simulink model "simulink_pi"  (R2018a)
settings: Solver=VariableStepAuto  StartTime=0.0  StopTime=500  RelTol=1e-3
values from neighbouring files (symbols this model uses):
  ae = 329.2  / fator    (= 5.48666666667)    [carregaDadosDoModelo.m]    (also in carregaDadosSimulacao.m = 5.4867)
  anp = 16.5    [carregaDadosSimulacao.m]
  av = 414.17 / fator    (= 6.90283333333)    [carregaDadosDoModelo.m]    (also in carregaDadosSimulacao.m = 6.9028)
  K = 0.36783    [carregaDados.m]    (also in carregaDadosDoModelo.m = 0.01332; carregaDadosSimulacao.m = 0.01)
  Kc = 1       * fator    (= 60)    [carregaDadosDoModelo.m]    (also in carregaDadosSimulacao.m = 2.5)
  Ke = 0.395   * fator    (= 23.7)    [carregaDadosDoModelo.m]    (also in carregaDadosSimulacao.m = 1.4)
  Ki = 13 * Kp    (= 1.56)    [carregaDados.m]    (also in carregaDadosSimulacao.m)
  Knp = 0.1    [carregaDadosSimulacao.m]
  Kp = 0.12    [carregaDados.m]    (also in carregaDadosSimulacao.m)
  Kpwm = 20    [carregaDadosSimulacao.m]
  Kr = 0.016835* fator    (= 1.0101)    [carregaDadosDoModelo.m]
  Ktp = 36.5    [carregaDadosSimulacao.m]
  Kv = 0.647   * fator    (= 38.82)    [carregaDadosDoModelo.m]    (also in carregaDadosSimulacao.m = 3.3)
  td = 0.065    [carregaDados.m]    (also in carregaDadosSimulacao.m = 5)
settings Model: Creator=alexa  LastModifiedBy=alexa

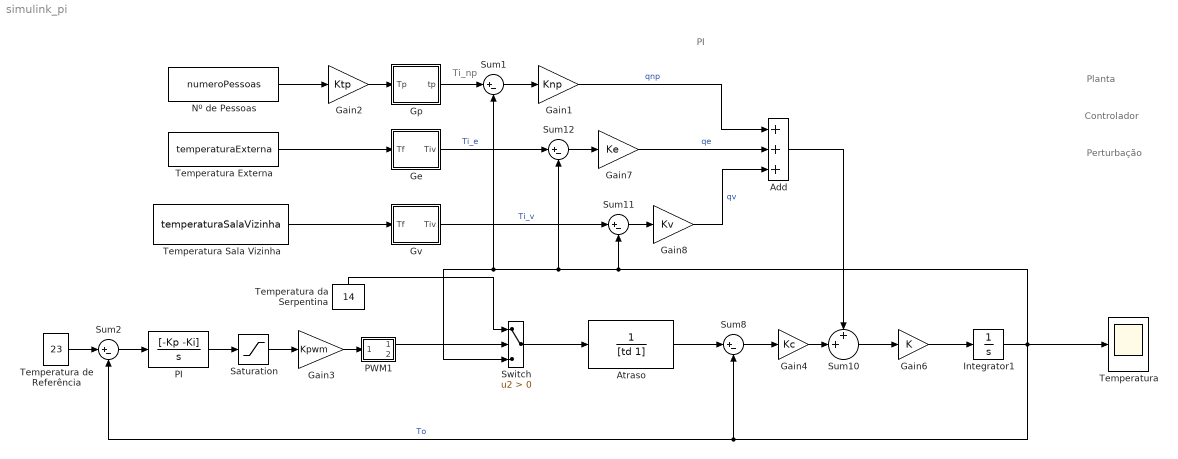
== system simulink_pi ==
  note: Planta
  note: Perturbação
  note: Ti_np
  note: Controlador
  note: PI
  Add : Sum  Inputs=+++
  Atraso : TransferFcn  Denominator=[td 1]
  Gain1 : Gain  Gain=Knp
  Gain2 : Gain  Gain=Ktp
  Gain3 : Gain  Gain=Kpwm
  Gain4 : Gain  Gain=Kc
  Gain6 : Gain  Gain=K
  Gain7 : Gain  Gain=Ke
  Gain8 : Gain  Gain=Kv
  Ge : Subsystem
  Gp : Subsystem
  Gv : Subsystem
  Integrator1 : Integrator  InitialCondition=24
  Nº de Pessoas : FromWorkspace  VariableName=numeroPessoas  SampleTime=1
  PI : TransferFcn  Numerator=[-Kp -Ki]  Denominator=[1 0]
  PWM1 : Subsystem  mask(Pulse Generator){period=1, amplitude=1, start=0}
      mask prompts: period "Period (secs):"; start "Start time:"
      mask help: Pulse Generator
      mask Help: Pulse generator which ensures pulse transitions are hit. Provides a vector of pulses when the height is entered as a vector.  Unmask to see how it works.
      mask Display: plot(0,0,100,100,[95,90,90,75,75,60,60,45,45,30,30,15,15,5],[25,25,75,75,25,25,75,75,25,25,75,75,25,25]);
  Saturation : Saturate  UpperLimit=0.05  LowerLimit=-0.05
  Sum{1..2,8,11..12} (5 alike) : Sum  Inputs=|+-
  Sum10 : Sum  Inputs=++|
  Switch : Switch  Criteria=u2 > Threshold
  Temperatura : Scope
  Temperatura da Serpentina : Constant  Value=14
  Temperatura de Referência : Constant  Value=23
  Temperatura Externa : FromWorkspace  VariableName=temperaturaExterna  SampleTime=1
  Temperatura Sala Vizinha : FromWorkspace  VariableName=temperaturaSalaVizinha  SampleTime=1
  wires:
  Sum12/1 -> Gain7/1
  Sum8/1 -> Gain4/1
  Gain7/1 -> Add/2  "qe"
  Gain2/1 -> Gp/1(Tp)
  Nº de Pessoas/1 -> Gain2/1
  Gp/1("tp ") -> Sum1/1
  Gain8/1 -> Add/3  "qv"
  Gain1/1 -> Add/1  "qnp"
  Temperatura Externa/1 -> Ge/1(Tf)
  Ge/1(Tiv) -> Sum12/1  "Ti_e"
  Integrator1/1 -> Temperatura/1, Sum8/2, Sum2/2, Switch/3, Sum1/2, Sum12/2, Sum11/2  "To"
  Temperatura da Serpentina/1 -> Switch/1
  Temperatura Sala Vizinha/1 -> Gv/1(Tf)
  Switch/1 -> Atraso/1
  Add/1 -> Sum10/1
  Gv/1(Tiv) -> Sum11/1  "Ti_v"
  Atraso/1 -> Sum8/1
  Sum11/1 -> Gain8/1
  Gain6/1 -> Integrator1/1
  Sum1/1 -> Gain1/1
  Sum10/1 -> Gain6/1
  Gain4/1 -> Sum10/2
  Temperatura de Referência/1 -> Sum2/1
  Sum2/1 -> PI/1
  PI/1 -> Saturation/1
  PWM1/1(Out1) -> Switch/2
  Saturation/1 -> Gain3/1
  Gain3/1 -> PWM1/1(In1)

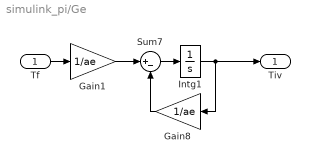
== system simulink_pi/Ge ==
  Tf : Inport
  Gain1 : Gain  Gain=1/ae
  Gain8 : Gain  Gain=1/ae
  Intg1 : Integrator  InitialCondition=30
  Sum7 : Sum  Inputs=|+-
  Tiv : Outport
  wires:
  Gain1/1 -> Sum7/1
  Tf/1 -> Gain1/1
  Gain8/1 -> Sum7/2
  Intg1/1 -> Tiv/1, Gain8/1
  Sum7/1 -> Intg1/1

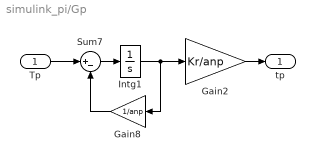
== system simulink_pi/Gp ==
  Tp : Inport
  Gain2 : Gain  Gain=Kr/anp
  Gain8 : Gain  Gain=1/anp
  Intg1 : Integrator
  Sum7 : Sum  Inputs=|+-
  "tp " : Outport
  wires:
  Gain2/1 -> "tp "/1
  Tp/1 -> Sum7/1
  Gain8/1 -> Sum7/2
  Intg1/1 -> Gain2/1, Gain8/1
  Sum7/1 -> Intg1/1

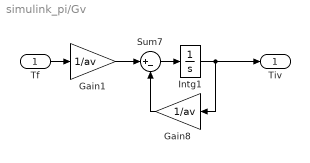
== system simulink_pi/Gv ==
  Tf : Inport
  Gain1 : Gain  Gain=1/av
  Gain8 : Gain  Gain=1/av
  Intg1 : Integrator  InitialCondition=30
  Sum7 : Sum  Inputs=|+-
  Tiv : Outport
  wires:
  Gain1/1 -> Sum7/1
  Tf/1 -> Gain1/1
  Gain8/1 -> Sum7/2
  Intg1/1 -> Tiv/1, Gain8/1
  Sum7/1 -> Intg1/1

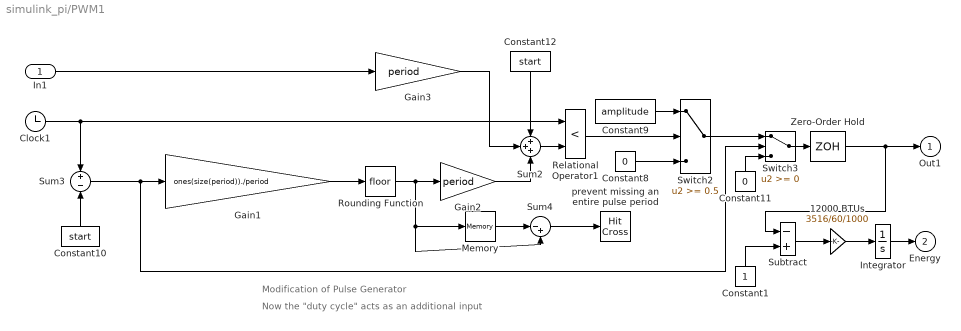
== system simulink_pi/PWM1 ==
  note: Now the "duty cycle" acts as an additional input
  note: Modification of Pulse Generator
  In1 : Inport
  12000 BTUs : Gain  Gain=3516/60/1000
  Clock1 : Clock
  Constant1 : Constant
  Constant10 : Constant  Value=start
  Constant11 : Constant  Value=0
  Constant12 : Constant  Value=start
  Constant8 : Constant  Value=0
  Constant9 : Constant  Value=amplitude
  Gain1 : Gain  Gain=ones(size(period))./period  SaturateOnIntegerOverflow=on  OutDataTypeStr=Inherit: Same as input  ParamDataTypeStr=Inherit: Same as input
  Gain2 : Gain  Gain=period  SaturateOnIntegerOverflow=on  OutDataTypeStr=Inherit: Same as input  ParamDataTypeStr=Inherit: Same as input
  Gain3 : Gain  Gain=period  SaturateOnIntegerOverflow=on  OutDataTypeStr=Inherit: Same as input  ParamDataTypeStr=Inherit: Same as input
  Integrator : Integrator
  Memory : Memory
  Relational Operator1 : RelationalOperator  Operator=<  RndMeth=Nearest  InputSameDT=on
  Rounding Function : Rounding
  Subtract : Sum  Inputs=-+
  Sum2 : Sum  Inputs=+++  SaturateOnIntegerOverflow=on  InputSameDT=on  OutDataTypeStr=Inherit: Same as first input
  Sum3 : Sum  Inputs=+-  SaturateOnIntegerOverflow=on  InputSameDT=on  OutDataTypeStr=Inherit: Same as first input
  Sum4 : Sum  Inputs=|-+  SaturateOnIntegerOverflow=on  InputSameDT=on  OutDataTypeStr=Inherit: Same as first input
  Switch2 : Switch  Threshold=0.5  SaturateOnIntegerOverflow=on  InputSameDT=on
  Switch3 : Switch  SaturateOnIntegerOverflow=on  InputSameDT=on
  Zero-Order Hold : ZeroOrderHold  SampleTime=.1
  prevent missing an entire pulse period : HitCross  HitCrossingOffset=1  ShowOutputPort=off
  Out1 : Outport
  Energy : Outport  Port=2
  wires:
  Gain3/1 -> Sum2/2
  Constant12/1 -> Sum2/1
  In1/1 -> Gain3/1
  Gain2/1 -> Sum2/3
  Constant10/1 -> Sum3/2
  Sum3/1 -> Gain1/1, Switch3/2
  Clock1/1 -> Relational Operator1/1, Sum3/1
  Sum2/1 -> Relational Operator1/2
  Gain1/1 -> Rounding Function/1
  Rounding Function/1 -> Sum4/2, Memory/1, Gain2/1
  Switch3/1 -> Zero-Order Hold/1
  Relational Operator1/1 -> Switch2/2
  Constant8/1 -> Switch2/3
  Constant9/1 -> Switch2/1
  Constant11/1 -> Switch3/3
  Switch2/1 -> Switch3/1
  Sum4/1 -> prevent missing an entire pulse period/1
  Memory/1 -> Sum4/1
  Zero-Order Hold/1 -> Out1/1, Subtract/1
  Integrator/1 -> Energy/1
  Constant1/1 -> Subtract/2
  12000 BTUs/1 -> Integrator/1
  Subtract/1 -> 12000 BTUs/1
